simulink model "acelerometro_mobile"  (R2025b)
settings: Solver=FixedStepDiscrete  StartTime=0.0  StopTime=inf  FixedStep=0.05  MaxStep=1/10000  RelTol=1e-3
StopFcn:
  | daqreset
settings Model: Creator=jesus  LastModifiedBy=jesus

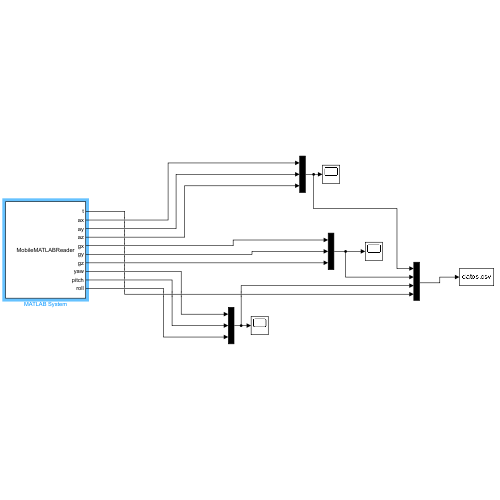
[thumbnail: Simulink's stored preview of the top-level diagram]
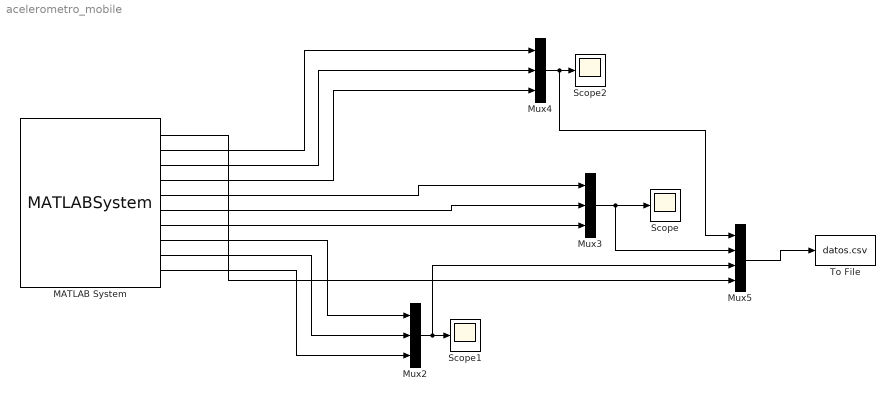
== system acelerometro_mobile ==
  MATLAB System : MATLABSystem  System=MobileMATLABReader  Rate=20  UseOrientation=true  WarnIfNoData=true  AutoReconnect=true  ReconnectPeriod=5  LogPurgePeriod=5  NoDataTimeout=8  ForceReconnectOnStale=true  CleanupBaseWorkspace=true  EnableDebugLog=true  DebugLogFile=mobilematlab_reader_debug.log  DebugSamplePeriod=2  JitterReportPeriod=5
      mask Type: MobileMATLABReader
  Mux2 : Mux  Inputs=3
  Mux3 : Mux  Inputs=3
  Mux4 : Mux  Inputs=3
  Mux5 : Mux
  Scope : Scope
      settings: ActiveDisplayYMinimum=-39.32824475  ActiveDisplayYMaximum=35.17557275
  Scope1 : Scope
      settings: ActiveDisplayYMinimum=-96.5392217532128  ActiveDisplayYMaximum=94.789638652650652
  Scope2 : Scope
      settings: ActiveDisplayYMinimum=-1  ActiveDisplayYMaximum=1  DataLoggingVariableName=ScopeData2
  To File : ToFile  Filename=datos.csv  MatrixName=senales
  wires:
  Mux5/1 -> To File/1
  Mux3/1 -> Mux5/2, Scope/1
  Mux2/1 -> Mux5/3, Scope1/1
  MATLAB System/8 -> Mux2/1
  MATLAB System/9 -> Mux2/2
  MATLAB System/10 -> Mux2/3
  MATLAB System/2 -> Mux4/1
  MATLAB System/3 -> Mux4/2
  MATLAB System/4 -> Mux4/3
  Mux4/1 -> Mux5/1, Scope2/1
  MATLAB System/5 -> Mux3/1
  MATLAB System/6 -> Mux3/2
  MATLAB System/7 -> Mux3/3
  MATLAB System/1 -> Mux5/4
